simulink model "HW2_PR3"  (R2019a)
settings: Solver=ode23s  StartTime=0.0  StopTime=100  RelTol=1e-3
InitFcn:
  | HW2_Q3_parameters
values from neighbouring files (symbols this model uses):
  c = 3    [HW2_P3_ab.m]    (also in HW2_Q1_parameters.m = 1; HW2_Q3_parameters.m)
  k = 5    [HW2_P3_ab.m]    (also in HW2_Q3_parameters.m)
  L1 = 1    [HW2_P3_ab.m]    (also in HW2_Q3_parameters.m)
  L2 = 2    [HW2_P3_ab.m]    (also in HW2_Q3_parameters.m)
  L3 = 2    [HW2_P3_ab.m]    (also in HW2_Q3_parameters.m)
  m = 10    [HW2_P3_ab.m]    (also in HW2_Q1_parameters.m = 2; HW2_Q3_parameters.m)
libraries: simulink_extras x1
settings Model: Creator=canba  LastModifiedBy=canba

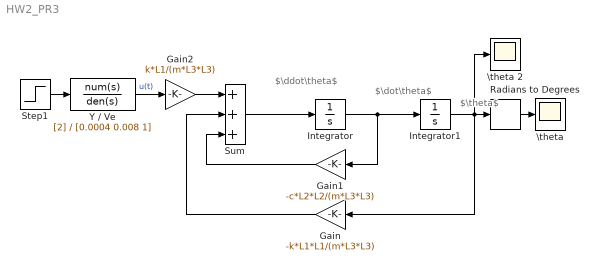
== system HW2_PR3 ==
  note: $\dot\theta$
  note: $\theta$
  note: $\ddot\theta$
  Gain : Gain  Gain=-k*L1*L1/(m*L3*L3)
  Gain1 : Gain  Gain=-c*L2*L2/(m*L3*L3)
  Gain2 : Gain  Gain=k*L1/(m*L3*L3)
  Integrator : Integrator
  Integrator1 : Integrator
  Radians to Degrees : simulink_extras/Transformations/Radians to Degrees
  Step1 : Step  Time=10  SampleTime=0
  Sum : Sum  Inputs=+++
  Y / Ve : TransferFcn  Numerator=[2]  Denominator=[0.0004 0.008 1]
  "\\theta " : Scope
  \theta 2 : Scope
  wires:
  Integrator/1 -> Gain1/1, Integrator1/1
  Sum/1 -> Integrator/1
  Integrator1/1 -> \theta 2/1, Gain/1, Radians to Degrees/1
  Gain/1 -> Sum/2
  Gain1/1 -> Sum/3
  Gain2/1 -> Sum/1
  Y / Ve/1 -> Gain2/1  "u(t)"
  Step1/1 -> Y / Ve/1
  Radians to Degrees/1 -> "\\theta "/1
